simulink model "Tune_Abstract_BDMotor_SDO"  (R2014a)
settings: Solver=ode45  StartTime=0.0  StopTime=2.5  MaxStep=1e-3  RelTol=1e-3
PostLoadFcn:
  | warning off Simulink:blocks:LegendInfoNA
  | load Ref_Data_BDMotor
  | open_system([bdroot '/Start Values']);
undefined symbols (not defined in the file or in its folder): q_scaling, slope, step_down
undefined symbols (not defined in the file): delay_periods, ramp_periods
libraries: simulink x2
Description:
  | Copyright 2014 The MathWorks, Inc.
settings Model: Creator=smiller  LastModifiedBy=psanghvi
settings DataIOCC: LimitDataPoints=off
settings DebuggingCC: UnderspecifiedInitializationDetection=Classic  StateNameClashWarn=warning

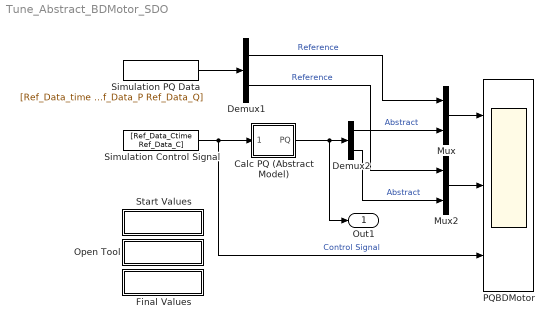
== system Tune_Abstract_BDMotor_SDO ==
  Calc PQ (Abstract Model) : Subsystem  mask{delay=round(delay_periods), ramp_dur=round(ramp_periods), step_down=step_down, slope=slope, q_scaling=q_scaling}
      mask prompts: delay "# Delay periods (10 ms)"; ramp_dur "# Ramp periods (10 ms)"; step_down "Peak max - steady state (W)"; slope "Ramp slope"; q_scaling "Q scale factor"
  Demux1 : Demux  Outputs=2
  Demux2 : Demux  Outputs=2
  Final Values : Subsystem
      settings: OpenFcn=|
      | delay_periods = 5;
      | ramp_periods = 45;
      | step_down = 452.3;
      | slope = 2432.3;
      | q_scaling = 0.2713;
      mask Display: disp('Final Values')
  Mux : Mux  Inputs=2
  Mux2 : Mux  Inputs=2
  Open Tool : Subsystem
      settings: OpenFcn=speload('Tune_Abstract_BDMotor_Project', 'Project - Tune_Abstract_BDMotor_Project', 'Param Est 1');
      mask Display: disp('Open Tool')
  PQBDMotor : Scope  NumInputPorts=3
      settings: ShowLegends=on  TimeRange=2.5  YMin=0~-50~-550  YMax=1500~400~550  SaveName=PQ_BDMotor  Decimation=10  SampleTime=10e-6
  Simulation Control Signal : FromWorkspace  VariableName=[Ref_Data_Ctime Ref_Data_C]  SampleTime=0
  Simulation PQ Data : FromWorkspace  VariableName=[Ref_Data_time Ref_Data_P Ref_Data_Q]  SampleTime=0
  Start Values : Subsystem
      settings: OpenFcn=|
      | delay_periods = 5;
      | ramp_periods = 45;
      | step_down = 250;
      | slope = 792;
      | q_scaling = 0.72;
      mask Display: disp('Start Values')
  Out1 : Outport
  wires:
  Simulation PQ Data/1 -> Demux1/1
  Simulation Control Signal/1 -> PQBDMotor/3, Calc PQ (Abstract Model)/1(Ctrl)  "Control Signal"
  Calc PQ (Abstract Model)/1(PQ) -> Out1/1, Demux2/1
  Demux2/1 -> Mux/2  "Abstract"
  Demux2/2 -> Mux2/2  "Abstract"
  Mux/1 -> PQBDMotor/1
  Mux2/1 -> PQBDMotor/2
  Demux1/1 -> Mux/1  "Reference"
  Demux1/2 -> Mux2/1  "Reference"

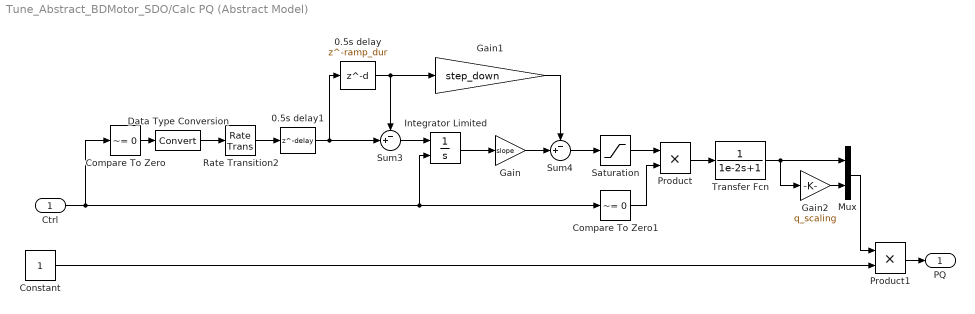
== system Tune_Abstract_BDMotor_SDO/Calc PQ (Abstract Model) ==
  Ctrl : Inport
  0.5s delay : Delay  DelayLength=ramp_dur  SampleTime=0.01
  0.5s delay1 : Delay  DelayLength=delay  SampleTime=0.01
  Compare To Zero : simulink/Logic and Bit Operations/Compare To Zero  relop=~=  OutDataTypeStr=boolean
  Compare To Zero1 : simulink/Logic and Bit Operations/Compare To Zero  relop=~=  OutDataTypeStr=boolean
  Constant : Constant
  Data Type Conversion : DataTypeConversion
  Gain : Gain  Gain=slope
  Gain1 : Gain  Gain=step_down
  Gain2 : Gain  Gain=q_scaling
  Integrator Limited : Integrator  ExternalReset=falling  LimitOutput=on  UpperSaturationLimit=1  LowerSaturationLimit=0
  Mux : Mux  Inputs=2
  Product : Product
  Product1 : Product
  Rate Transition2 : RateTransition  OutPortSampleTime=0.01
  Saturation : Saturate  UpperLimit=1160  LowerLimit=0
  Sum3 : Sum  Inputs=-+|  SaturateOnIntegerOverflow=on  InputSameDT=on  OutDataTypeStr=Inherit: Same as first input
  Sum4 : Sum  Inputs=-+|  SaturateOnIntegerOverflow=on  InputSameDT=on  OutDataTypeStr=Inherit: Same as first input
  Transfer Fcn : TransferFcn  Denominator=[1e-2 1]
  PQ : Outport
  wires:
  Product1/1 -> PQ/1
  Constant/1 -> Product1/2
  0.5s delay1/1 -> 0.5s delay/1, Sum3/2
  Ctrl/1 -> Compare To Zero/1, Compare To Zero1/1, Integrator Limited/2
  Mux/1 -> Product1/1
  Gain2/1 -> Mux/2
  Transfer Fcn/1 -> Mux/1, Gain2/1
  Compare To Zero/1 -> Data Type Conversion/1
  Integrator Limited/1 -> Gain/1
  Data Type Conversion/1 -> Rate Transition2/1
  Gain/1 -> Sum4/2
  Rate Transition2/1 -> 0.5s delay1/1
  Sum3/1 -> Integrator Limited/1
  Product/1 -> Transfer Fcn/1
  Gain1/1 -> Sum4/1
  0.5s delay/1 -> Sum3/1, Gain1/1
  Sum4/1 -> Saturation/1
  Saturation/1 -> Product/1
  Compare To Zero1/1 -> Product/2

== system Tune_Abstract_BDMotor_SDO/Final Values ==

== system Tune_Abstract_BDMotor_SDO/Open Tool ==

== system Tune_Abstract_BDMotor_SDO/Start Values ==
